simulink model "simQ2"  (R2018b)
settings: Solver=VariableStepAuto  StartTime=0.0  StopTime=T  RelTol=1e-3
values from neighbouring files (symbols this model uses):
  Kd = 1    [MAIN_hw6.m]
  Kp = 200    [MAIN_hw6.m]
  X0 = [0; 0]    [MAIN_hw6.m]
undefined symbols (not defined in the file or in its folder): controller, fcnODE
settings Model: Creator=Erivelton  LastModifiedBy=Erivelton

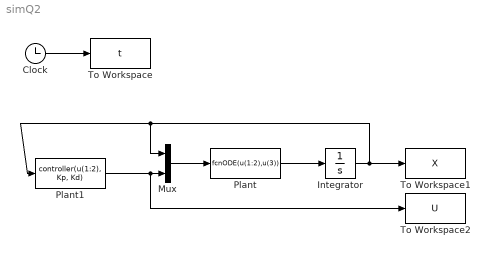
== system simQ2 ==
  Clock : Clock
  Integrator : Integrator  InitialCondition=X0
  Mux : Mux  Inputs=2
  Plant : MATLABFcn  MATLABFcn=fcnODE(u(1:2),u(3))
  Plant1 : MATLABFcn  MATLABFcn=controller(u(1:2), Kp, Kd)
  To Workspace : ToWorkspace  VariableName=t  SampleTime=-1
  To Workspace1 : ToWorkspace  VariableName=X  SampleTime=-1
  To Workspace2 : ToWorkspace  VariableName=U  SampleTime=-1
  wires:
  Mux/1 -> Plant/1
  Plant/1 -> Integrator/1
  Integrator/1 -> To Workspace1/1, Plant1/1, Mux/1
  Plant1/1 -> To Workspace2/1, Mux/2
  Clock/1 -> To Workspace/1
